simulink model "audio_fn"  (R2019b)
settings: Solver=VariableStepAuto  StartTime=0.0  StopTime=60  RelTol=1e-3
libraries: simulink_extras x1, dspsnks4 x1, dspvision x1
settings Model: Creator=ARES  LastModifiedBy=ARES

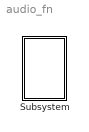
== system audio_fn ==
  Subsystem : Subsystem

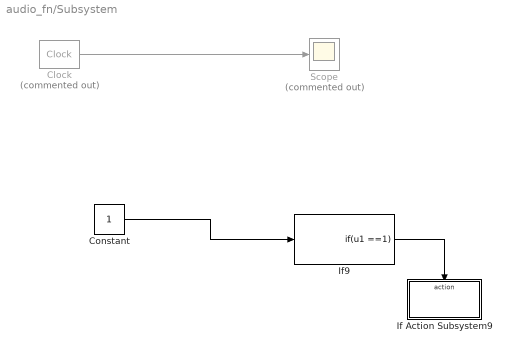
== system audio_fn/Subsystem ==
  Clock : simulink_extras/Flip Flops/Clock  Commented=on  period=10
  Constant : Constant
  If Action Subsystem9 : Subsystem  TreatAsAtomicUnit=on
  If9 : If  IfExpression=u1 ==1  ShowElse=off
  Scope : Scope  Commented=on
  wires:
  If9/1 -> If Action Subsystem9/Action
  Clock/1 -> Scope/1
  Constant/1 -> If9/1

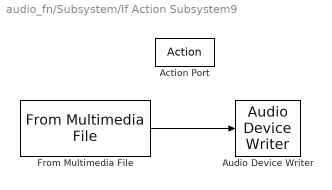
== system audio_fn/Subsystem/If Action Subsystem9 ==
  Action Port : ActionPort  ActionPortLabel=if(u1 ==1)
  Audio Device Writer : dspsnks4/Audio Device Writer  Driver=DirectSound  Device=Headphones (Beats Solo� Stereo)  InheritSampleRate=on  SampleRate=44100  BitDepth=16-bit integer  BufferSize=4096  NumBuffers=10  DefaultOutputChannelMapping=on  OutputChannelMapping=1:2  OutputNumUnderrunSamples=off  DriverIdx=1  DeviceWarnFlag=''
  From Multimedia File : dspvision/From Multimedia File  inputFilename=C:\Users\ARES\Documents\ARES Simulation SR\ALARMS\Alarm_Bad.wav  readRange=[1 Inf]  loop=on  numPlays=1  outputStreams=Audio only  videoDataType=single  audioDataType=double  inheritSampleTime=on  userDefinedSampleTime=1/30  noAudioOutput=off  isIntensityVideo=off  fourcc=RGB  colorVideoFormat=Separate color signals  outputEOF=off  dataOrg=Column-major  audioFrameSize=1024  computeAudioFrameSize=off  outSamplingMode=Sample based
      settings: SourceProductName=DSP System Toolbox  SourceProductBaseCode=DS
  wires:
  From Multimedia File/1 -> Audio Device Writer/1
